simulink model "Sistem1"  (R2024a)
settings: Solver=ode1be  StartTime=0.0  StopTime=250  FixedStep=0.01  MaxStep=0.1  RelTol=1e-3
values from neighbouring files (symbols this model uses):
  de_count = Simulink.Parameter(de_count_local)    [valoriMamdaniTest.m]
  de_points = Simulink.Parameter(de_points_local)    [valoriMamdaniTest.m]
  e_count = Simulink.Parameter(e_count_local)    [valoriMamdaniTest.m]
  e_points = Simulink.Parameter(e_points_local)    [valoriMamdaniTest.m]
  gamma = Simulink.Parameter(gamma_local)    [valoriMamdaniTest.m]
settings Model: Creator=Monica  LastModifiedBy=Monica
settings SolverCC: ZeroCrossControl=EnableAll

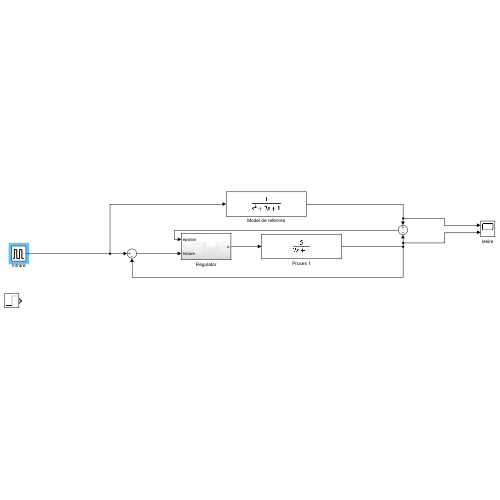
[thumbnail: Simulink's stored preview of the top-level diagram]
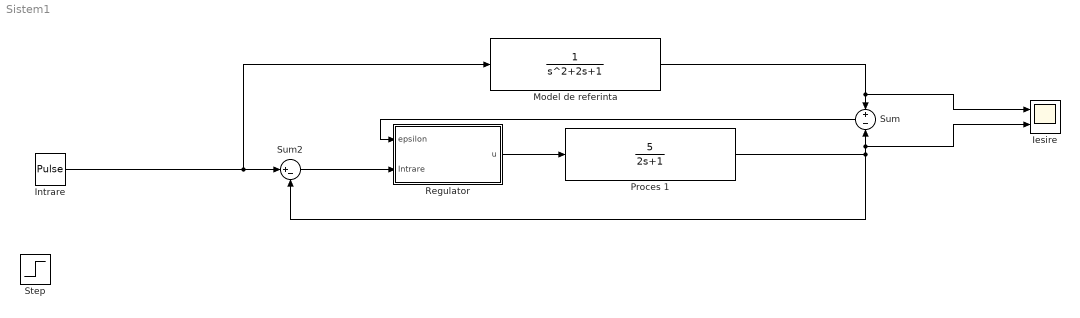
== system Sistem1 ==
  Iesire : Scope  NumInputPorts=2
  Intrare : DiscretePulseGenerator  PulseType=Time based  Period=40  PulseWidth=50
  Model de referinta : TransferFcn
  Proces 1 : TransferFcn  Numerator=[5]  Denominator=[2 1]
  Regulator : Subsystem
  Step : Step  SampleTime=0
  Sum : Sum  Inputs=+|-
  Sum2 : Sum  Inputs=|+-
  wires:
  Model de referinta/1 -> Iesire/1, Sum/1
  Proces 1/1 -> Iesire/2, Sum/2, Sum2/2
  Regulator/1(u) -> Proces 1/1
  Sum2/1 -> Regulator/2(Intrare)
  Intrare/1 -> Model de referinta/1, Sum2/1
  Sum/1 -> Regulator/1(epsilon)

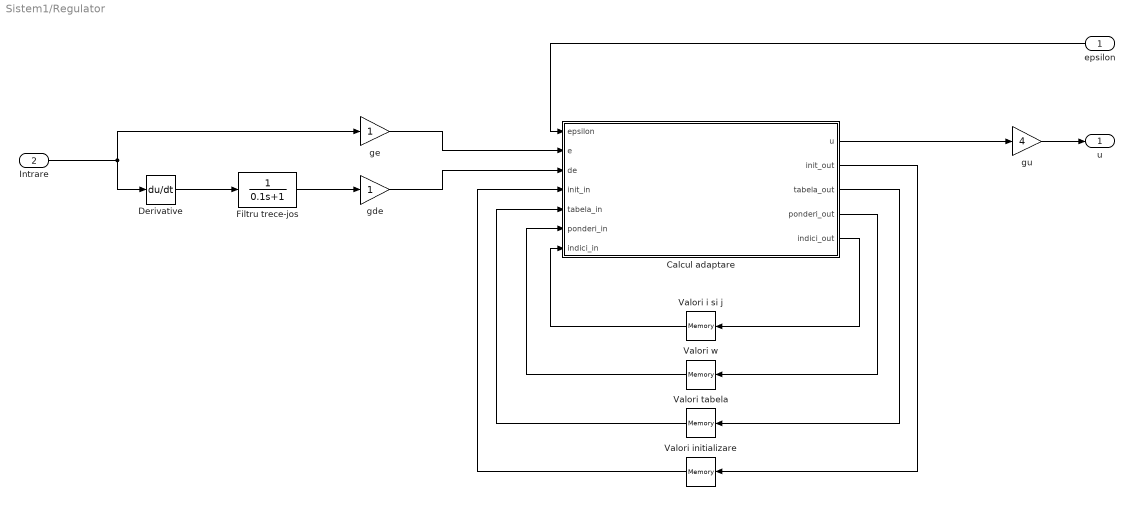
== system Sistem1/Regulator ==
  epsilon : Inport
  Intrare : Inport  Port=2
  Calcul adaptare : MATLAB Function  TreatAsAtomicUnit=on
  Derivative : Derivative
  Filtru trece-jos : TransferFcn  Denominator=[0.1 1]
  Valori i si j : Memory  InheritSampleTime=on
  Valori initializare : Memory  InheritSampleTime=on
  Valori tabela : Memory  InheritSampleTime=on
  Valori w : Memory  InheritSampleTime=on
  gde : Gain
  ge : Gain
  gu : Gain  Gain=4
  u : Outport
  wires:
  Calcul adaptare/2(init_out) -> Valori initializare/1
  Valori initializare/1 -> Calcul adaptare/4(init_in)
  Valori tabela/1 -> Calcul adaptare/5(tabela_in)
  Intrare/1 -> Derivative/1, ge/1
  Derivative/1 -> Filtru trece-jos/1
  Valori w/1 -> Calcul adaptare/6(ponderi_in)
  epsilon/1 -> Calcul adaptare/1(epsilon)
  ge/1 -> Calcul adaptare/2(e)
  gde/1 -> Calcul adaptare/3(de)
  gu/1 -> u/1
  Calcul adaptare/5(indici_out) -> Valori i si j/1
  Valori i si j/1 -> Calcul adaptare/7(indici_in)
  Calcul adaptare/3(tabela_out) -> Valori tabela/1
  Calcul adaptare/1(u) -> gu/1
  Calcul adaptare/4(ponderi_out) -> Valori w/1
  Filtru trece-jos/1 -> gde/1

== matlab function Sistem1/Regulator/Calcul adaptare ==
  data: epsilon input; u output; e input; de input; init_in input; init_out output; tabela_in input size=[1,dim_tabela]; tabela_out output; ponderi_out output; ponderi_in input size=[1,4]; indici_in input size=[1,2]; indici_out output; e_count parameter; de_count parameter; e_points parameter; de_points parameter; gamma parameter
function [u, init_out, tabela_out, ponderi_out, indici_out] = TabelaDeDecizieMamdani(epsilon, e, de, init_in, tabela_in, ponderi_in, indici_in, e_count, de_count, e_points, de_points, gamma)
    clc

    % Utilizarea parametrilor Simulink 
    gamma = gamma; % Rata de adaptare

    e_count = e_count;  
    de_count = de_count;  
    e_points = e_points;  
    de_points = de_points; 

    % Prealocare memorie 
    init_out = init_in;
    tabela_out = tabela_in;

    if init_in == 0
        init_out = 1;
        tabela_out(:) = 0;
    end    

    % Adaptare tabela
    i_a = max(1, min(indici_in(1), e_count));
    j_a = max(1, min(indici_in(2), de_count));
    index = (i_a - 1) * de_count + j_a;

    if i_a < e_count && j_a < de_count
        % Interior (4 valori)
        tabela_out(index) = tabela_in(index) + gamma * ponderi_in(1) * epsilon;
        tabela_out(index + de_count) = tabela_in(index + de_count) + gamma * ponderi_in(2) * epsilon;
        tabela_out(index + 1) = tabela_in(index + 1) + gamma * ponderi_in(3) * epsilon;
        tabela_out(index + de_count + 1) = tabela_in(index + de_count + 1) + gamma * ponderi_in(4) * epsilon;
    elseif i_a == e_count && j_a == de_count
        % Colt dreapta-jos (1 valoare)
        tabela_out(index) = tabela_in(index) + gamma * epsilon;
    elseif i_a == e_count
        % Margine dreapta (2 valori)
        tabela_out(index) = tabela_in(index) + gamma * 0.5 * epsilon;
        tabela_out(index + 1) = tabela_in(index + 1) + gamma * 0.5 * epsilon;
    elseif j_a == de_count
        % Margine jos (2 valori)
        tabela_out(index) = tabela_in(index) + gamma * 0.5 * epsilon;
        tabela_out(index + de_count) = tabela_in(index + de_count) + gamma * 0.5 * epsilon;
    else
        % Colt stânga-sus 
        tabela_out(index) = tabela_in(index) + gamma * epsilon;
    end

    % Calcul ponderi si u
    [~, i] = min(abs(e_points - e));
    [~, j] = min(abs(de_points - de));
    
    indici_out = [i, j];
    index = (i - 1) * de_count + j;

    if i < e_count && j < de_count
        % Interior (4 valori)
        w_ij = (e_points(i + 1) - e) * (de_points(j + 1) - de) / ((e_points(i + 1) - e_points(i)) * (de_points(j + 1) - de_points(j)));
        w_i1j = (e - e_points(i)) * (de_points(j + 1) - de) / ((e_points(i + 1) - e_points(i)) * (de_points(j + 1) - de_points(j)));
        w_ij1 = (e_points(i + 1) - e) * (de - de_points(j)) / ((e_points(i + 1) - e_points(i)) * (de_points(j + 1) - de_points(j)));
        w_i1j1 = (e - e_points(i)) * (de - de_points(j)) / ((e_points(i + 1) - e_points(i)) * (de_points(j + 1) - de_points(j)));
        
        ponderi_out = [w_ij, w_i1j, w_ij1, w_i1j1];
        u = w_ij * tabela_out(index) + w_i1j * tabela_out(index + de_count) + w_ij1 * tabela_out(index + 1) + w_i1j1 * tabela_out(index + de_count + 1);
    elseif i == e_count && j == de_count
        % Colt dreapta-jos
        ponderi_out = [1, 0, 0, 0];
        u = tabela_out(index);
    elseif i == e_count
        % Margine dreapta 
        w1 = (de_points(j + 1) - de) / (de_points(j + 1) - de_points(j));
        w2 = 1 - w1;
        
        ponderi_out = [w1, w2, 0, 0];
        u = w1 * tabela_out(index) + w2 * tabela_out(index + 1);
    elseif j == de_count
        % Margine jos 
        w1 = (e_points(i + 1) - e) / (e_points(i + 1) - e_points(i));
        w2 = 1 - w1;
        
        ponderi_out = [w1, 0, w2, 0];
        u = w1 * tabela_out(index) + w2 * tabela_out(index + de_count);
    else
        % Colt stanga-sus 
        ponderi_out = [1, 0, 0, 0];
        u = tabela_out(index);
    end

    % Stocarea in workspace a tabelei Mamdani
    assignin("base", "MamdaniFinal", tabela_out);
end
